simulink model "modelzbiornikow"  (R2015a)
settings: Solver=ode3  StartTime=0.0  StopTime=500  FixedStep=0.01  RelTol=1e-3
values from neighbouring files (symbols this model uses):
  A = l1(1:3,1:3)    [linearyzacja.m]    (also in lqrr.m = [-a1*C1*h1^(a1-1)/c*w, 0, 0;a1*C2*h1^(a1-1)/S1, -a2*C2*h2^(a)
  a = 35    [lqrr.m]
  B = l1(1:3,4)    [linearyzacja.m]    (also in lqrr.m = [1/(c*w);0;0])
  b = 37    [lqrr.m]
  C = eye(3)    [linearyzacja.m]    (also in lqrr.m)
  c = 10    [lqrr.m]
  D = zeros(3,1)    [linearyzacja.m]    (also in lqrr.m = [0;0;0])
  h2max = 35    [lqrr.m]
  K = lqr(A,B,Q,r)    [regulator_LQR.m]
  R = 36.4    [lqrr.m]
  w = 5    [lqrr.m]
undefined symbols (not defined in the file or in its folder): a1, a2, a3, C1, C2, C3, h1, h2, h3, q
libraries: simulink x4
settings Model: Creator=Ziger  LastModifiedBy=Student

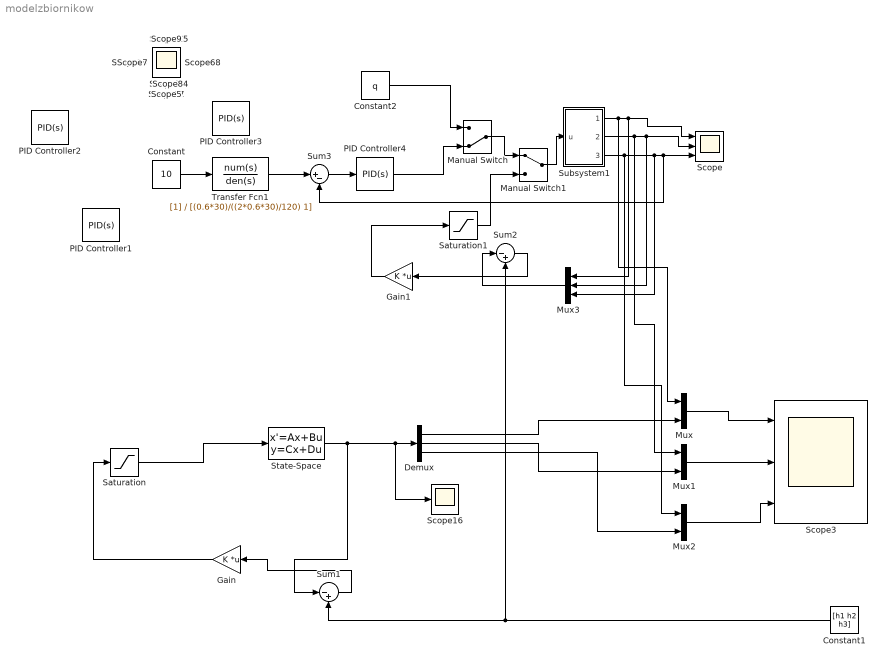
== system modelzbiornikow ==
  Constant : Constant  Value=10
  Constant1 : Constant  Value=[h1 h2 h3]
  Constant2 : Constant  Value=q
  Demux : Demux  Outputs=3
  Gain : Gain  Gain=K  Multiplication=Matrix(K*u)
  Gain1 : Gain  Gain=K  Multiplication=Matrix(K*u)
  Manual Switch : ManualSwitch  CurrentSetting=0
  Manual Switch1 : ManualSwitch
  Mux : Mux  Inputs=2
  Mux1 : Mux  Inputs=2
  Mux2 : Mux  Inputs=2
  Mux3 : Mux  Inputs=3
  PID Controller1 : simulink/Continuous/PID Controller  Controller=PID  TimeDomain=Continuous-time  SampleTime=-1  IntegratorMethod=Forward Euler  FilterMethod=Forward Euler  Form=Parallel  UseFilter=on  ControllerParametersSource=internal  P=19.1234820716003  I=0.160486934444709  D=564.398521740036  N=1.87487265962734  InitialConditionSource=internal  InitialConditionForIntegrator=0  InitialConditionForFilter=0  ExternalReset=none  LimitOutput=on  UpperSaturationLimit=160  LowerSaturationLimit=0  LinearizeAsGain=on  AntiWindupMode=none  Kb=1  TrackingMode=off  Kt=1  PParamMin=[]  PParamMax=[]  IParamMin=[]  IParamMax=[]  DParamMin=[]  DParamMax=[]  NParamMin=[]  NParamMax=[]  KbParamMin=[]  KbParamMax=[]  KtParamMin=[]  KtParamMax=[]  POutMin=[]  POutMax=[]  IOutMin=[]  IOutMax=[]  DOutMin=[]  DOutMax=[]  NOutMin=[]  NOutMax=[]  KbOutMin=[]  KbOutMax=[]  KtOutMin=[]  KtOutMax=[]  IntegratorOutMin=[]  IntegratorOutMax=[]  FilterOutMin=[]  FilterOutMax=[]  SumOutMin=[]  SumOutMax=[]  SumI1OutMin=[]  SumI1OutMax=[]  SumI2OutMin=[]  SumI2OutMax=[]  SumI3OutMin=[]  SumI3OutMax=[]  SumDOutMin=[]  SumDOutMax=[]  SaturationOutMin=[]  SaturationOutMax=[]  IntegratorContinuousStateAttributes=''  IntegratorStateMustResolveToSignalObject=off  IntegratorRTWStateStorageClass=Auto  FilterContinuousStateAttributes=''  FilterStateMustResolveToSignalObject=off  FilterRTWStateStorageClass=Auto  DifferentiatorICPrevScaledInput=0  DifferentiatorOutMin=[]  DifferentiatorOutMax=[]
  PID Controller2 : simulink/Continuous/PID Controller  Controller=PID  TimeDomain=Continuous-time  SampleTime=-1  IntegratorMethod=Forward Euler  FilterMethod=Forward Euler  Form=Parallel  UseFilter=on  ControllerParametersSource=internal  P=32.2909472864139  I=0.180231567349232  D=1433.5067168856  N=2.90923724524028  InitialConditionSource=internal  InitialConditionForIntegrator=0  InitialConditionForFilter=0  ExternalReset=none  LimitOutput=on  UpperSaturationLimit=160  LowerSaturationLimit=0  LinearizeAsGain=on  AntiWindupMode=none  Kb=1  TrackingMode=off  Kt=1  PParamMin=[]  PParamMax=[]  IParamMin=[]  IParamMax=[]  DParamMin=[]  DParamMax=[]  NParamMin=[]  NParamMax=[]  KbParamMin=[]  KbParamMax=[]  KtParamMin=[]  KtParamMax=[]  POutMin=[]  POutMax=[]  IOutMin=[]  IOutMax=[]  DOutMin=[]  DOutMax=[]  NOutMin=[]  NOutMax=[]  KbOutMin=[]  KbOutMax=[]  KtOutMin=[]  KtOutMax=[]  IntegratorOutMin=[]  IntegratorOutMax=[]  FilterOutMin=[]  FilterOutMax=[]  SumOutMin=[]  SumOutMax=[]  SumI1OutMin=[]  SumI1OutMax=[]  SumI2OutMin=[]  SumI2OutMax=[]  SumI3OutMin=[]  SumI3OutMax=[]  SumDOutMin=[]  SumDOutMax=[]  SaturationOutMin=[]  SaturationOutMax=[]  IntegratorContinuousStateAttributes=''  IntegratorStateMustResolveToSignalObject=off  IntegratorRTWStateStorageClass=Auto  FilterContinuousStateAttributes=''  FilterStateMustResolveToSignalObject=off  FilterRTWStateStorageClass=Auto  DifferentiatorICPrevScaledInput=0  DifferentiatorOutMin=[]  DifferentiatorOutMax=[]
  PID Controller3 : simulink/Continuous/PID Controller  Controller=PID  TimeDomain=Continuous-time  SampleTime=-1  IntegratorMethod=Forward Euler  FilterMethod=Forward Euler  Form=Parallel  UseFilter=on  ControllerParametersSource=internal  P=0.6*45  I=(2*0.6*45)/76  D=(45*76)/8  N=1  InitialConditionSource=internal  InitialConditionForIntegrator=0  InitialConditionForFilter=0  ExternalReset=none  LimitOutput=on  UpperSaturationLimit=inf  LowerSaturationLimit=0  LinearizeAsGain=on  AntiWindupMode=none  Kb=1  TrackingMode=off  Kt=1  PParamMin=[]  PParamMax=[]  IParamMin=[]  IParamMax=[]  DParamMin=[]  DParamMax=[]  NParamMin=[]  NParamMax=[]  KbParamMin=[]  KbParamMax=[]  KtParamMin=[]  KtParamMax=[]  POutMin=[]  POutMax=[]  IOutMin=[]  IOutMax=[]  DOutMin=[]  DOutMax=[]  NOutMin=[]  NOutMax=[]  KbOutMin=[]  KbOutMax=[]  KtOutMin=[]  KtOutMax=[]  IntegratorOutMin=[]  IntegratorOutMax=[]  FilterOutMin=[]  FilterOutMax=[]  SumOutMin=[]  SumOutMax=[]  SumI1OutMin=[]  SumI1OutMax=[]  SumI2OutMin=[]  SumI2OutMax=[]  SumI3OutMin=[]  SumI3OutMax=[]  SumDOutMin=[]  SumDOutMax=[]  SaturationOutMin=[]  SaturationOutMax=[]  IntegratorContinuousStateAttributes=''  IntegratorStateMustResolveToSignalObject=off  IntegratorRTWStateStorageClass=Auto  FilterContinuousStateAttributes=''  FilterStateMustResolveToSignalObject=off  FilterRTWStateStorageClass=Auto  DifferentiatorICPrevScaledInput=0  DifferentiatorOutMin=[]  DifferentiatorOutMax=[]
  PID Controller4 : simulink/Continuous/PID Controller  Controller=PID  TimeDomain=Continuous-time  SampleTime=-1  IntegratorMethod=Forward Euler  FilterMethod=Forward Euler  Form=Parallel  UseFilter=on  ControllerParametersSource=internal  P=0.6*30  I=(2*0.6*30)/120  D=(30*120)/8  N=1  InitialConditionSource=internal  InitialConditionForIntegrator=0  InitialConditionForFilter=0  ExternalReset=none  LimitOutput=on  UpperSaturationLimit=inf  LowerSaturationLimit=0  LinearizeAsGain=on  AntiWindupMode=none  Kb=1  TrackingMode=off  Kt=1  PParamMin=[]  PParamMax=[]  IParamMin=[]  IParamMax=[]  DParamMin=[]  DParamMax=[]  NParamMin=[]  NParamMax=[]  KbParamMin=[]  KbParamMax=[]  KtParamMin=[]  KtParamMax=[]  POutMin=[]  POutMax=[]  IOutMin=[]  IOutMax=[]  DOutMin=[]  DOutMax=[]  NOutMin=[]  NOutMax=[]  KbOutMin=[]  KbOutMax=[]  KtOutMin=[]  KtOutMax=[]  IntegratorOutMin=[]  IntegratorOutMax=[]  FilterOutMin=[]  FilterOutMax=[]  SumOutMin=[]  SumOutMax=[]  SumI1OutMin=[]  SumI1OutMax=[]  SumI2OutMin=[]  SumI2OutMax=[]  SumI3OutMin=[]  SumI3OutMax=[]  SumDOutMin=[]  SumDOutMax=[]  SaturationOutMin=[]  SaturationOutMax=[]  IntegratorContinuousStateAttributes=''  IntegratorStateMustResolveToSignalObject=off  IntegratorRTWStateStorageClass=Auto  FilterContinuousStateAttributes=''  FilterStateMustResolveToSignalObject=off  FilterRTWStateStorageClass=Auto  DifferentiatorICPrevScaledInput=0  DifferentiatorOutMin=[]  DifferentiatorOutMax=[]
  Saturation : Saturate  UpperLimit=160  LowerLimit=0
  Saturation1 : Saturate  UpperLimit=160  LowerLimit=0
  Scope : Scope  NumInputPorts=3
      settings: TimeRange=500  YMin=0~0~0  YMax=40~6~12  SaveName=zbiorniki
  Scope{1..2,4..19} (18 alike) : Scope
      Scope16 settings: YMin=3  YMax=9  SaveName=ScopeData14
      Scope10 settings: SaveName=ScopeData8
      Scope11 settings: SaveName=ScopeData9
      Scope12 settings: SaveName=ScopeData10
      Scope13 settings: SaveName=ScopeData11
      Scope14 settings: SaveName=ScopeData12
      Scope15 settings: SaveName=ScopeData13
      Scope17 settings: SaveName=ScopeData15
      Scope18 settings: SaveName=ScopeData16
      Scope19 settings: SaveName=ScopeData17
      Scope4 settings: SaveName=ScopeData7
      Scope5 settings: SaveName=ScopeData2
      Scope6 settings: SaveName=ScopeData3
      Scope7 settings: SaveName=ScopeData4
      Scope8 settings: TimeRange=450  SaveName=ScopeData5
      Scope9 settings: SaveName=ScopeData6
  Scope3 : Scope  NumInputPorts=3
      settings: TimeRange=500  YMin=-50~-2~5.5  YMax=250~9~11.5  SaveName=zbiorniki_apro
  State-Space : StateSpace  A=A  B=B  C=C  D=D  X0=0
  Subsystem1 : Subsystem
  Sum1 : Sum  Inputs=|-+
  Sum2 : Sum  Inputs=|-+
  Sum3 : Sum  Inputs=|+-
  Transfer Fcn1 : TransferFcn  Denominator=[(0.6*30)/((2*0.6*30)/120) 1]
  wires:
  Subsystem1/1(h1out) -> Mux/1, Mux3/1, Scope/1
  Subsystem1/2("h2out ") -> Mux1/1, Mux3/2, Scope/2
  Subsystem1/3("h3out ") -> Mux2/1, Mux3/3, Sum3/2, Scope/3
  Mux/1 -> Scope3/1
  Mux1/1 -> Scope3/2
  Mux2/1 -> Scope3/3
  Constant2/1 -> Manual Switch/1
  Sum3/1 -> PID Controller4/1
  PID Controller4/1 -> Manual Switch/2
  Demux/1 -> Mux/2
  Demux/2 -> Mux1/2
  Demux/3 -> Mux2/2
  State-Space/1 -> Sum1/1, Scope16/1, Demux/1
  Constant1/1 -> Sum1/2, Sum2/2
  Sum1/1 -> Gain/1
  Gain/1 -> Saturation/1
  Saturation/1 -> State-Space/1
  Mux3/1 -> Sum2/1
  Sum2/1 -> Gain1/1
  Gain1/1 -> Saturation1/1
  Manual Switch/1 -> Manual Switch1/1
  Saturation1/1 -> Manual Switch1/2
  Manual Switch1/1 -> Subsystem1/1(u)
  Constant/1 -> Transfer Fcn1/1
  Transfer Fcn1/1 -> Sum3/1

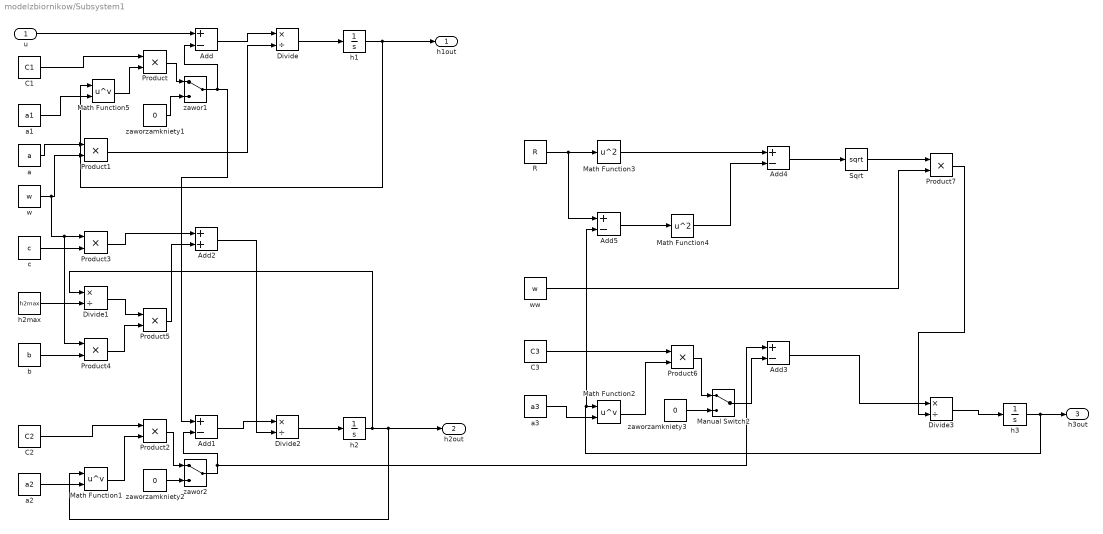
== system modelzbiornikow/Subsystem1 ==
  u : Inport
  Add{,1,3..5} (5 alike) : Sum  Inputs=+-
  Add2 : Sum
  C1 : Constant  Value=C1
  C2 : Constant  Value=C2
  C3 : Constant  Value=C3
  Divide{,1..3} (4 alike) : Product  Inputs=*/
  Manual Switch2 : ManualSwitch
  Math Function1 : Math  Operator=pow  SaturateOnIntegerOverflow=on
  Math Function2 : Math  Operator=pow  SaturateOnIntegerOverflow=on
  Math Function3 : Math  Operator=square  SaturateOnIntegerOverflow=on
  Math Function4 : Math  Operator=square  SaturateOnIntegerOverflow=on
  Math Function5 : Math  Operator=pow  SaturateOnIntegerOverflow=on
  Product{,1..7} (8 alike) : Product
  R : Constant  Value=R
  Sqrt : Sqrt  SaturateOnIntegerOverflow=on
  a : Constant  Value=a
  a1 : Constant  Value=a1
  a2 : Constant  Value=a2
  a3 : Constant  Value=a3
  b : Constant  Value=b
  c : Constant  Value=c
  h1 : Integrator  LimitOutput=on  UpperSaturationLimit=35  LowerSaturationLimit=0
  h2 : Integrator  LimitOutput=on  UpperSaturationLimit=35  LowerSaturationLimit=0
  h2max : Constant  Value=h2max
  h3 : Integrator  InitialCondition=2  LimitOutput=on  UpperSaturationLimit=35  LowerSaturationLimit=0
  w : Constant  Value=w
  ww : Constant  Value=w
  "zawor1 " : ManualSwitch
  "zawor2 " : ManualSwitch
  zaworzamkniety1 : Constant  Value=0
  zaworzamkniety2 : Constant  Value=0
  zaworzamkniety3 : Constant  Value=0
  h1out : Outport
  "h2out " : Outport  Port=2
  "h3out " : Outport  Port=3
  wires:
  h1/1 -> Math Function5/1, h1out/1
  h2/1 -> Divide1/1, "h2out "/1, Math Function1/1
  Math Function1/1 -> Product2/2
  u/1 -> Add/1
  Add/1 -> Divide/1
  Product/1 -> "zawor1 "/1
  C1/1 -> Product/1
  a/1 -> Product1/1
  Product4/1 -> Product5/2
  Product1/1 -> Divide/2
  h2max/1 -> Divide1/2
  C2/1 -> Product2/1
  w/1 -> Product4/1, Product3/1, Product1/2
  Divide2/1 -> h2/1
  Product7/1 -> Divide3/2
  Add2/1 -> Divide2/2
  Divide1/1 -> Product5/1
  a2/1 -> Math Function1/2
  Product5/1 -> Add2/2
  Add3/1 -> Divide3/1
  R/1 -> Add5/1, Math Function3/1
  h3/1 -> "h3out "/1, Add5/2, Math Function2/1
  Math Function3/1 -> Add4/1
  Add4/1 -> Sqrt/1
  Divide3/1 -> h3/1
  Sqrt/1 -> Product7/1
  Math Function2/1 -> Product6/2
  b/1 -> Product4/2
  Add5/1 -> Math Function4/1
  a3/1 -> Math Function2/2
  Product3/1 -> Add2/1
  C3/1 -> Product6/1
  ww/1 -> Product7/2
  Math Function4/1 -> Add4/2
  Add1/1 -> Divide2/1
  c/1 -> Product3/2
  zaworzamkniety1/1 -> "zawor1 "/2
  "zawor1 "/1 -> Add1/1, Add/2
  Product2/1 -> "zawor2 "/1
  zaworzamkniety2/1 -> "zawor2 "/2
  "zawor2 "/1 -> Add3/1, Add1/2
  Product6/1 -> Manual Switch2/1
  zaworzamkniety3/1 -> Manual Switch2/2
  Manual Switch2/1 -> Add3/2
  Divide/1 -> h1/1
  a1/1 -> Math Function5/2
  Math Function5/1 -> Product/2
